simulink library "INT_InjVlv_BlkSht"  (R2016b)
settings: Solver=VariableStepAuto  StartTime=0.0  StopTime=10.0  RelTol=1e-3
settings Model: Creator=zhoutinglin  LastModifiedBy=zhoutinglin

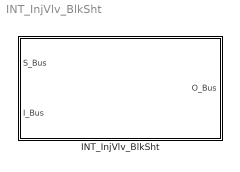
== system INT_InjVlv_BlkSht ==
  INT_InjVlv_BlkSht : Subsystem

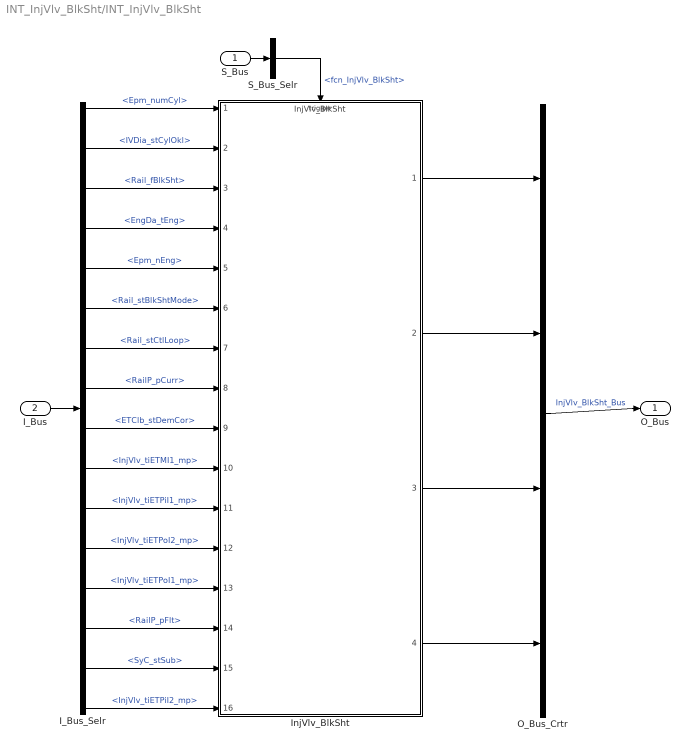
== system INT_InjVlv_BlkSht/INT_InjVlv_BlkSht ==
  S_Bus : Inport
  I_Bus : Inport  Port=2
  I_Bus_Selr : BusSelector  OutputSignals=Epm_numCyl,IVDia_stCylOkl,Rail_fBlkSht,EngDa_tEng,Epm_nEng,Rail_stBlkShtMode,Rail_stCtlLoop,RailP_pCurr,ETClb_stDemCor,InjVlv_tiETMI1_mp,InjVlv_tiETPiI1_mp,InjVlv_tiETPoI2_mp,InjVlv_tiETPoI1_mp,RailP_pFlt,SyC_stSub,InjVlv_tiETPiI2_mp
  InjVlv_BlkSht : ModelReference  ModelNameDialog=InjVlv_BlkSht  SimulationMode=Normal  ModelReferenceVersion=1.63  TriggerPortName=function  TriggerPortTriggerType=function-call  TriggerPortStatesWhenEnabling=held
  O_Bus_Crtr : BusCreator  Inputs=4
  S_Bus_Selr : BusSelector  OutputSignals=fcn_InjVlv_BlkSht
  O_Bus : Outport
  wires:
  S_Bus_Selr/1 -> InjVlv_BlkSht/Trigger  "<fcn_InjVlv_BlkSht>"
  S_Bus/1 -> S_Bus_Selr/1
  I_Bus/1 -> I_Bus_Selr/1
  I_Bus_Selr/1 -> InjVlv_BlkSht/1  "<Epm_numCyl>"
  I_Bus_Selr/2 -> InjVlv_BlkSht/2  "<IVDia_stCylOkl>"
  I_Bus_Selr/3 -> InjVlv_BlkSht/3  "<Rail_fBlkSht>"
  I_Bus_Selr/4 -> InjVlv_BlkSht/4  "<EngDa_tEng>"
  I_Bus_Selr/5 -> InjVlv_BlkSht/5  "<Epm_nEng>"
  I_Bus_Selr/6 -> InjVlv_BlkSht/6  "<Rail_stBlkShtMode>"
  I_Bus_Selr/7 -> InjVlv_BlkSht/7  "<Rail_stCtlLoop>"
  I_Bus_Selr/8 -> InjVlv_BlkSht/8  "<RailP_pCurr>"
  I_Bus_Selr/9 -> InjVlv_BlkSht/9  "<ETClb_stDemCor>"
  I_Bus_Selr/10 -> InjVlv_BlkSht/10  "<InjVlv_tiETMI1_mp>"
  I_Bus_Selr/11 -> InjVlv_BlkSht/11  "<InjVlv_tiETPiI1_mp>"
  I_Bus_Selr/12 -> InjVlv_BlkSht/12  "<InjVlv_tiETPoI2_mp>"
  I_Bus_Selr/13 -> InjVlv_BlkSht/13  "<InjVlv_tiETPoI1_mp>"
  I_Bus_Selr/14 -> InjVlv_BlkSht/14  "<RailP_pFlt>"
  I_Bus_Selr/15 -> InjVlv_BlkSht/15  "<SyC_stSub>"
  I_Bus_Selr/16 -> InjVlv_BlkSht/16  "<InjVlv_tiETPiI2_mp>"
  O_Bus_Crtr/1 -> O_Bus/1  "InjVlv_BlkSht_Bus"
  InjVlv_BlkSht/1 -> O_Bus_Crtr/1
  InjVlv_BlkSht/2 -> O_Bus_Crtr/2
  InjVlv_BlkSht/3 -> O_Bus_Crtr/3
  InjVlv_BlkSht/4 -> O_Bus_Crtr/4
